simulink model "gm_sampleModel1666_2_sub"  (R2023a)
settings: Solver=VariableStepAuto  StartTime=0.0  StopTime=10.0  RelTol=1e-3
libraries: simulink x2
settings Model: Creator=user1  LastModifiedBy=user1
settings OptimizationCC: BlockReduction=off  ConditionallyExecuteInputs=off
settings DebuggingCC: InheritedTsInSrcMsg=none

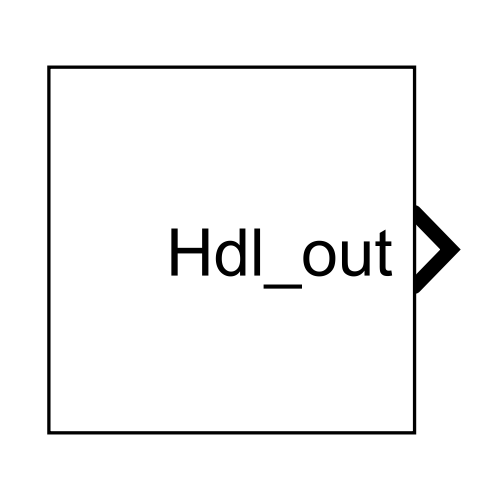
[thumbnail: Simulink's stored preview of the top-level diagram]
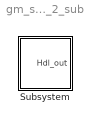
== system gm_sampleModel1666_2_sub ==
  Subsystem : Subsystem

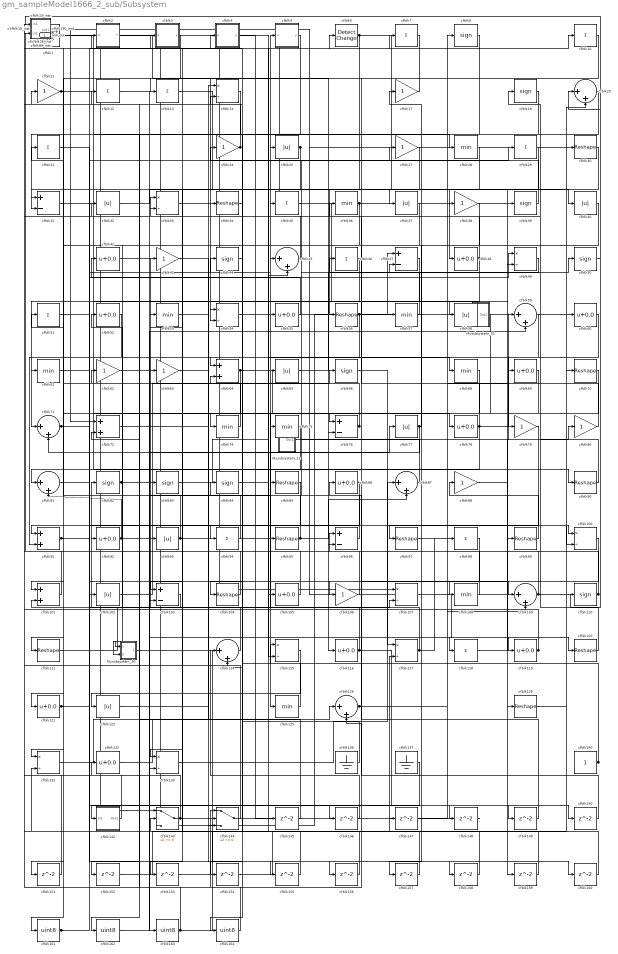
== system gm_sampleModel1666_2_sub/Subsystem ==
  Mysubsystem_12 : Subsystem
  Mysubsystem_30 : Subsystem
  Mysubsystem_31 : Subsystem
  cfblk1 : simulink/Logic and Bit Operations/Extract Bits  bitsToExtract=Upper half  numBits=8  bitIdxRange=[0 7]  outScalingMode=Preserve fixed-point scaling
      settings: LibrarySourceBlock=|
      | hdlsllib/Logic and Bit
      | Operations/Extract Bits
  cfblk{7,10,12..13,21,29,35,46,51,94,98,118} (12 alike) : Sum  Inputs=+  OutDataTypeStr=uint8
  cfblk{14,33,49,54,100,107,115,117,131,133} (10 alike) : Product  Inputs=*/  OutDataTypeStr=uint8  RndMeth=Zero  SaturateOnIntegerOverflow=on
  cfblk{64,72,91,101} (4 alike) : Sum  OutDataTypeStr=uint8
  cfblk{25,32,37,40,58,65,77,93,102,122} (10 alike) : Abs  OutDataTypeStr=uint8  SaturateOnIntegerOverflow=off
  cfblk{31,47,76,96,103} (5 alike) : Sum  Inputs=+-  OutDataTypeStr=uint8
  cfblk{30,34,56,70,85,90,95,97,99,104,111,120,129} (13 alike) : Reshape
  cfblk{42,48,52,55,60,69,78,86,92,105,116,119,121,132} (14 alike) : Bias  Bias=0.0  SaturateOnIntegerOverflow=off
  cfblk{11,17,24,27,38,43,62..63,79..80,88,106} (12 alike) : Gain  OutDataTypeStr=uint8
  cfblk{28,36,53,57,61,68,74..75,108,125} (10 alike) : MinMax  OutDataTypeStr=uint8
  cfblk{20,45,59,71,81,87,109,114,126} (9 alike) : Sum  Inputs=|++  OutDataTypeStr=uint8
  cfblk{8,19,39,44,50,66,82..84,110} (10 alike) : Signum
  cfblk112_inst : Subsystem
  cfblk113_inst : Subsystem
  cfblk124_inst : Subsystem
  cfblk128_inst : Subsystem
  cfblk130_inst : Subsystem
  cfblk136 : Ground
  cfblk137 : Ground
  cfblk140 : Constant  OutDataTypeStr=uint8  SampleTime=-1
  cfblk142 : Subsystem
  cfblk143 : Switch  OutDataTypeStr=uint8  SaturateOnIntegerOverflow=off  InputSameDT=off
  cfblk144 : Switch  OutDataTypeStr=uint8  SaturateOnIntegerOverflow=off  InputSameDT=off
  cfblk{145..160} (16 alike) : Delay  SampleTime=1
  cfblk15_inst : Subsystem
  cfblk{161..164} (4 alike) : DataTypeConversion  OutDataTypeStr=uint8  SaturateOnIntegerOverflow=off  RndMeth=Floor
  cfblk16_inst : Subsystem
  cfblk2 : Subsystem  mask(Detect Rise Positive){vinit=double(0), InputProcessing=Elements as channels (sample based), OutDataTypeStr=uint8}
      mask prompts: vinit "Simulink:masks:InitialCondition_MP"; InputProcessing "Simulink:masks:InputProcessing_MP"; OutDataTypeStr "Simulink:masks:OutputDataType_MP"
      mask help: Simulink:masks:DetectRisePositive_MD
      mask init:
      | InputProcessing = 'Elements as channels (sample based)';
      | OutDataTypeStr = 'uint8';
      | vinit = double(0);
      mask TypeOptions InputProcessing: Simulink:masks:ColumnsAsChannelsFrameBased | Simulink:masks:ElementsAsChannelsSampleBased
      mask TypeOptions OutDataTypeStr: Simulink:masks:uint8 | Simulink:masks:boolean
      mask Display: fprintf('U > 0\n&  NOT\nU/z > 0')
  cfblk26_inst : Subsystem
  cfblk3 : Subsystem  mask(Compare To Zero){relop=<=, OutDataTypeStr=uint8, ZeroCross=on}
      mask prompts: relop "Simulink:masks:Operator_MP"; OutDataTypeStr "Simulink:masks:OutputDataType_MP"; ZeroCross "Simulink:masks:EnableZerocrossingDetection_MP"
      mask help: Simulink:masks:CompareToZero_MD
      mask init:
      | OutDataTypeStr = 'uint8';
      | ZeroCross = 'on';
      | blkName = 'sampleModel1666_2_sub/Subsystem/cfblk3';
      | relop = '<=';
      | setValue = 'fixdt(0, 8)';
      mask TypeOptions relop: == | ~= | < | <= | >= | >
      mask TypeOptions OutDataTypeStr: Simulink:masks:uint8 | Simulink:masks:boolean
      mask Callback ZeroCross: sl('zeroCrossEnable', gcbh);
      mask Display: disp([relop,' 0'])
  cfblk4 : Subsystem  mask(Compare To Constant){relop=<=, const=double(3), OutDataTypeStr=uint8, ZeroCross=on}
      mask prompts: relop "Simulink:masks:Operator_MP"; const "Simulink:masks:ConstantValue_MP"; OutDataTypeStr "Simulink:masks:OutputDataType_MP"; ZeroCross "Simulink:masks:EnableZerocrossingDetection_MP"
      mask help: Simulink:masks:CompareToConstant_MD
      mask init:
      | OutDataTypeStr = 'uint8';
      | ZeroCross = 'on';
      | blkName = 'sampleModel1666_2_sub/Subsystem/cfblk4';
      | const = double(3);
      | const_str = '3.0';
      | const_val = double(3);
      | relop = '<=';
      | setValue = 'fixdt(0, 8)';
      | str = '<= 3';
      mask TypeOptions relop: == | ~= | < | <= | >= | >
      mask TypeOptions OutDataTypeStr: Simulink:masks:uint8 | Simulink:masks:boolean
      mask Callback ZeroCross: sl('zeroCrossEnable', gcbh);
      mask Display: disp(str)
  cfblk5 : Subsystem  mask(Compare To Constant){relop=<=, const=double(3), OutDataTypeStr=uint8, ZeroCross=on}
      mask prompts: relop "Simulink:masks:Operator_MP"; const "Simulink:masks:ConstantValue_MP"; OutDataTypeStr "Simulink:masks:OutputDataType_MP"; ZeroCross "Simulink:masks:EnableZerocrossingDetection_MP"
      mask help: Simulink:masks:CompareToConstant_MD
      mask init:
      | OutDataTypeStr = 'uint8';
      | ZeroCross = 'on';
      | blkName = 'sampleModel1666_2_sub/Subsystem/cfblk5';
      | const = double(3);
      | const_str = '3.0';
      | const_val = double(3);
      | relop = '<=';
      | setValue = 'fixdt(0, 8)';
      | str = '<= 3';
      mask TypeOptions relop: == | ~= | < | <= | >= | >
      mask TypeOptions OutDataTypeStr: Simulink:masks:uint8 | Simulink:masks:boolean
      mask Callback ZeroCross: sl('zeroCrossEnable', gcbh);
      mask Display: disp(str)
  cfblk6 : simulink/Logic and Bit Operations/Detect Change  vinit=0  OutDataTypeStr=uint8
      settings: LibrarySourceBlock=|
      | hdlsllib/Logic and Bit
      | Operations/Detect
      | Change
  cfblk89_inst : Subsystem
  Hdl_out : Outport  OutDataTypeStr=uint8  SampleTime=1
  wires:
  Mysubsystem_12/1(Out1) -> cfblk59/1
  Mysubsystem_30/1(Out1) -> cfblk156/1
  Mysubsystem_31/1(Out1) -> cfblk125/1
  cfblk1/1 -> cfblk58/1, cfblk28/1
  cfblk10/1 -> cfblk54/2
  cfblk100/1 -> cfblk144/1
  cfblk101/1 -> cfblk130_inst/2(in2)
  cfblk102/1 -> cfblk66/1
  cfblk103/1 -> cfblk82/1
  cfblk104/1 -> cfblk43/1
  cfblk105/1 -> cfblk4/1(u)
  cfblk106/1 -> cfblk33/1
  cfblk107/1 -> cfblk119/1
  cfblk108/1 -> cfblk96/1
  cfblk109/1 -> cfblk128_inst/1(in1), cfblk5/1(u)
  cfblk11/1 -> cfblk90/1, cfblk76/1
  cfblk110/1 -> cfblk112_inst/2(in2), cfblk62/1
  cfblk111/1 -> cfblk93/1
  cfblk112_inst/1(out1) -> cfblk145/1
  cfblk113_inst/1(out1) -> cfblk30/1
  cfblk114/1 -> cfblk53/1
  cfblk115/1 -> cfblk122/1
  cfblk116/1 -> cfblk55/1, cfblk150/1
  cfblk117/1 -> cfblk52/1, cfblk98/1
  cfblk118/1 -> cfblk80/1
  cfblk119/1 -> cfblk124_inst/1(in1), cfblk63/1
  cfblk12/1 -> cfblk163/1
  cfblk120/1 -> cfblk33/2
  cfblk121/1 -> cfblk149/1, cfblk148/1, cfblk107/2
  cfblk122/1 -> cfblk34/1
  cfblk124_inst/1(out1) -> cfblk57/1
  cfblk125/1 -> cfblk115/1
  cfblk126/1 -> cfblk86/1, cfblk8/1
  cfblk128_inst/1(out1) -> cfblk110/1, Hdl_out/1
  cfblk129/1 -> cfblk70/1
  cfblk13/1 -> cfblk56/1
  cfblk130_inst/1(out1) -> cfblk143/1
  cfblk131/1 -> cfblk14/1
  cfblk132/1 -> cfblk126/1
  cfblk133/1 -> cfblk87/1
  cfblk136/1 -> cfblk14/2
  cfblk137/1 -> cfblk142/1(In1)
  cfblk14/1 -> cfblk162/1
  cfblk140/1 -> cfblk92/1, cfblk128_inst/2(in2), cfblk2/1(U)
  cfblk142/1(Out1) -> cfblk15_inst/1(in1)
  cfblk143/1 -> cfblk83/1, cfblk132/1
  cfblk144/1 -> cfblk89_inst/1(in1)
  cfblk145/1 -> cfblk72/2
  cfblk146/1 -> cfblk114/1
  cfblk147/1 -> cfblk109/2
  cfblk148/1 -> cfblk1/1
  cfblk149/1 -> cfblk101/2
  cfblk15_inst/1(out1) -> cfblk72/1
  cfblk150/1 -> cfblk126/2
  cfblk151/1 -> cfblk130_inst/1(in1)
  cfblk152/1 -> cfblk45/2
  cfblk153/1 -> cfblk117/2
  cfblk154/1 -> cfblk20/2
  cfblk155/1 -> cfblk64/2
  cfblk156/1 -> cfblk113_inst/1(in1)
  cfblk157/1 -> cfblk103/2
  cfblk158/1 -> cfblk26_inst/2(in2)
  cfblk159/1 -> cfblk143/2
  cfblk16_inst/1(out1) -> cfblk107/1
  cfblk160/1 -> cfblk131/2
  cfblk161/1 -> cfblk44/1, cfblk49/1
  cfblk162/1 -> cfblk85/1
  cfblk163/1 -> cfblk113_inst/2(in2), cfblk147/1
  cfblk164/1 -> cfblk12/1
  cfblk17/1 -> cfblk13/1
  cfblk19/1 -> cfblk31/2
  cfblk2/1(Y) -> cfblk76/2
  cfblk20/1 -> cfblk121/1
  cfblk21/1 -> cfblk102/1
  cfblk24/1 -> cfblk15_inst/2(in2), cfblk124_inst/2(in2)
  cfblk25/1 -> cfblk153/1, cfblk152/1
  cfblk26_inst/1(out1) -> cfblk95/1, cfblk39/1, cfblk16_inst/1(in1)
  cfblk27/1 -> cfblk37/1
  cfblk28/1 -> cfblk115/2
  cfblk29/1 -> cfblk48/1
  cfblk3/1(y) -> cfblk101/1
  cfblk30/1 -> cfblk91/1
  cfblk31/1 -> cfblk116/1
  cfblk32/1 -> cfblk38/1
  cfblk33/1 -> cfblk40/1
  cfblk34/1 -> cfblk74/1
  cfblk35/1 -> cfblk129/1
  cfblk36/1 -> cfblk111/1, Mysubsystem_30/1(In1)
  cfblk37/1 -> cfblk114/2
  cfblk38/1 -> cfblk54/1
  cfblk39/1 -> cfblk24/1
  cfblk4/1(y) -> cfblk106/1
  cfblk40/1 -> cfblk97/1
  cfblk42/1 -> cfblk75/1
  cfblk43/1 -> cfblk144/2
  cfblk44/1 -> cfblk164/1
  cfblk45/1 -> cfblk21/1
  cfblk46/1 -> cfblk71/1
  cfblk47/1 -> cfblk133/1
  cfblk48/1 -> cfblk89_inst/2(in2), cfblk154/1
  cfblk49/1 -> cfblk47/2
  cfblk5/1(y) -> cfblk104/1
  cfblk50/1 -> cfblk20/1
  cfblk51/1 -> cfblk29/1
  cfblk52/1 -> cfblk61/1
  cfblk53/1 -> cfblk120/1
  cfblk54/1 -> cfblk68/1
  cfblk55/1 -> cfblk42/1
  cfblk56/1 -> cfblk47/1, Mysubsystem_30/2(In2)
  cfblk57/1 -> cfblk32/1
  cfblk58/1 -> cfblk60/1, cfblk143/3
  cfblk59/1 -> cfblk79/1
  cfblk6/1 -> cfblk99/1, cfblk64/1, cfblk49/2
  cfblk60/1 -> cfblk91/2
  cfblk61/1 -> cfblk109/1
  cfblk62/1 -> cfblk78/1
  cfblk63/1 -> cfblk158/1
  cfblk64/1 -> cfblk96/2, cfblk144/3
  cfblk65/1 -> cfblk50/1
  cfblk66/1 -> cfblk117/1
  cfblk68/1 -> cfblk103/1
  cfblk69/1 -> cfblk81/1
  cfblk7/1 -> cfblk146/1
  cfblk70/1 -> cfblk151/1
  cfblk71/1 -> cfblk100/1, cfblk7/1
  cfblk72/1 -> cfblk27/1
  cfblk74/1 -> cfblk3/1(u)
  cfblk75/1 -> cfblk133/2
  cfblk76/1 -> cfblk25/1, cfblk51/1
  cfblk77/1 -> cfblk71/2, cfblk17/1
  cfblk78/1 -> cfblk131/1, cfblk100/2, cfblk46/1
  cfblk79/1 -> cfblk157/1
  cfblk8/1 -> cfblk31/1
  cfblk80/1 -> cfblk36/1
  cfblk81/1 -> cfblk45/1
  cfblk82/1 -> cfblk59/2, cfblk118/1
  cfblk83/1 -> cfblk10/1
  cfblk84/1 -> cfblk105/1
  cfblk85/1 -> cfblk161/1
  cfblk86/1 -> cfblk94/1
  cfblk87/1 -> cfblk35/1
  cfblk88/1 -> cfblk159/1
  cfblk89_inst/1(out1) -> cfblk112_inst/1(in1)
  cfblk90/1 -> cfblk19/1
  cfblk91/1 -> cfblk160/1, cfblk6/1
  cfblk92/1 -> cfblk84/1, cfblk81/2, cfblk77/1
  cfblk93/1 -> cfblk155/1, cfblk11/1
  cfblk94/1 -> cfblk26_inst/1(in1)
  cfblk95/1 -> cfblk87/2, cfblk16_inst/2(in2)
  cfblk96/1 -> cfblk65/1
  cfblk97/1 -> cfblk69/1
  cfblk98/1 -> cfblk108/1
  cfblk99/1 -> cfblk88/1

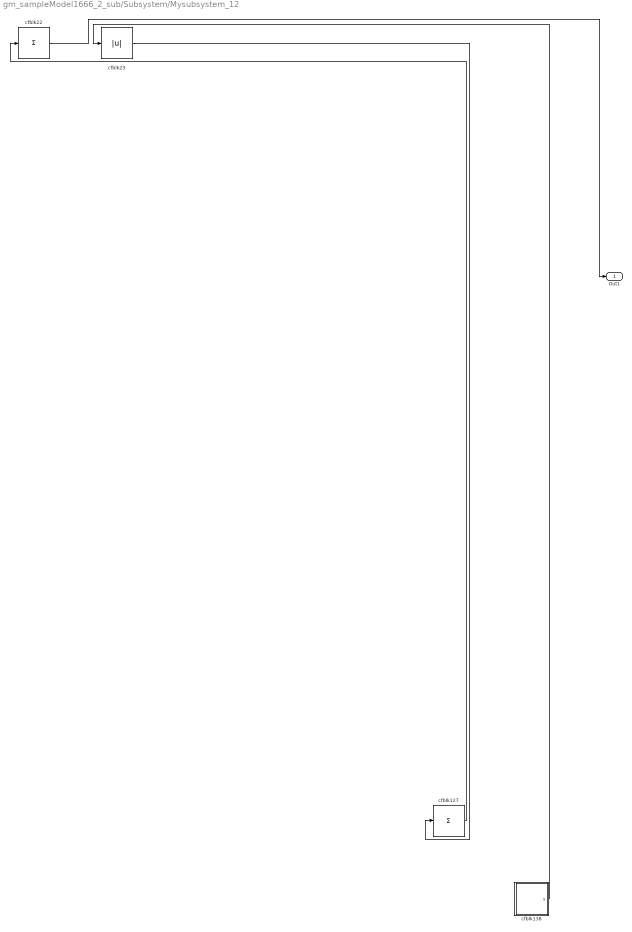
== system gm_sampleModel1666_2_sub/Subsystem/Mysubsystem_12 ==
  cfblk127 : Sum  Inputs=+
  cfblk138 : Subsystem  mask(Counter Free-Running){NumBits=double(16), tsamp=double(-1)}
      mask prompts: NumBits "Simulink:masks:NumberOfBits_MP"; tsamp "Simulink:masks:SampleTime_MP"
      mask help: Simulink:masks:CounterFreeRunning_MD
  cfblk22 : Sum  Inputs=+
  cfblk23 : Abs  SaturateOnIntegerOverflow=off
  Out1 : Outport  SampleTime=1
  wires:
  cfblk127/1 -> cfblk22/1
  cfblk138/1(y) -> cfblk23/1
  cfblk22/1 -> Out1/1
  cfblk23/1 -> cfblk127/1

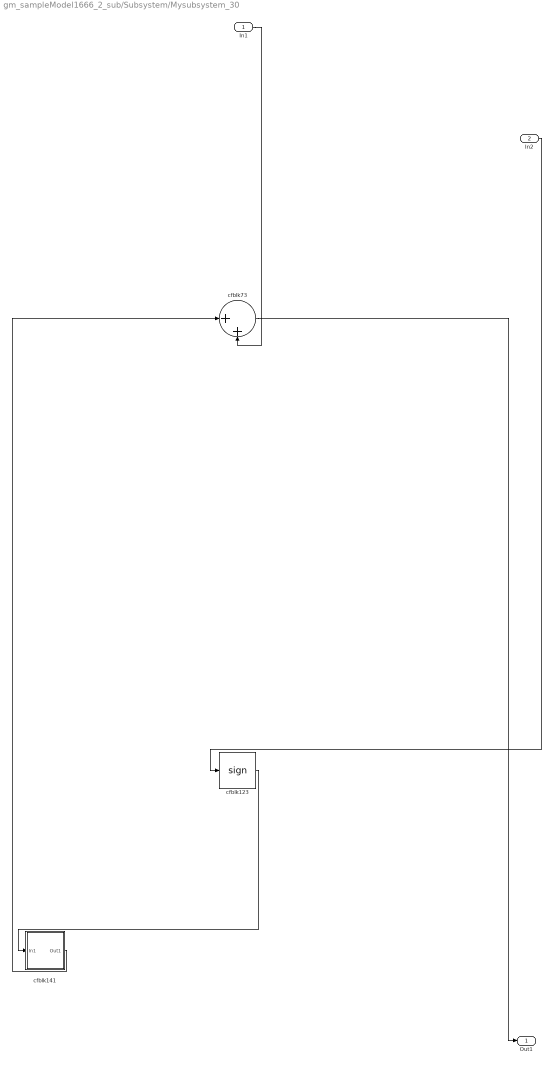
== system gm_sampleModel1666_2_sub/Subsystem/Mysubsystem_30 ==
  In1 : Inport  OutDataTypeStr=uint8  PortDimensions=1  SampleTime=1
  In2 : Inport  Port=2  OutDataTypeStr=uint8  PortDimensions=1  SampleTime=1
  cfblk123 : Signum
  cfblk141 : Subsystem
  cfblk73 : Sum  Inputs=|++
  Out1 : Outport  SampleTime=1
  wires:
  In1/1 -> cfblk73/2
  In2/1 -> cfblk123/1
  cfblk123/1 -> cfblk141/1(In1)
  cfblk141/1(Out1) -> cfblk73/1
  cfblk73/1 -> Out1/1

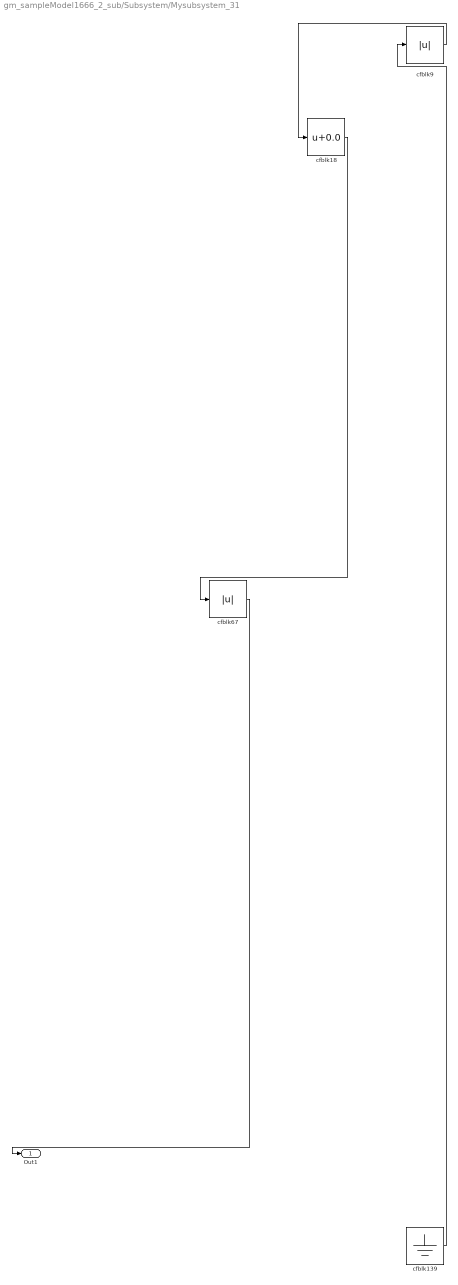
== system gm_sampleModel1666_2_sub/Subsystem/Mysubsystem_31 ==
  cfblk139 : Ground
  cfblk18 : Bias  Bias=0.0  SaturateOnIntegerOverflow=off
  cfblk67 : Abs  SaturateOnIntegerOverflow=off
  cfblk9 : Abs  SaturateOnIntegerOverflow=off
  Out1 : Outport  SampleTime=1
  wires:
  cfblk139/1 -> cfblk9/1
  cfblk18/1 -> cfblk67/1
  cfblk67/1 -> Out1/1
  cfblk9/1 -> cfblk18/1

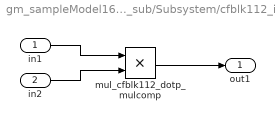
== system gm_sampleModel1666_2_sub/Subsystem/cfblk112_inst ==
  in1 : Inport  OutDataTypeStr=uint8  SampleTime=1
  in2 : Inport  Port=2  OutDataTypeStr=uint8  SampleTime=1
  mul_cfblk112_dotp_mulcomp : Product  Inputs=**  OutDataTypeStr=uint8  SampleTime=1
  out1 : Outport  OutDataTypeStr=uint8  SampleTime=1
  wires:
  in1/1 -> mul_cfblk112_dotp_mulcomp/1
  in2/1 -> mul_cfblk112_dotp_mulcomp/2
  mul_cfblk112_dotp_mulcomp/1 -> out1/1

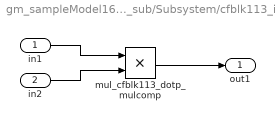
== system gm_sampleModel1666_2_sub/Subsystem/cfblk113_inst ==
  in1 : Inport  OutDataTypeStr=uint8  SampleTime=1
  in2 : Inport  Port=2  OutDataTypeStr=uint8  SampleTime=1
  mul_cfblk113_dotp_mulcomp : Product  Inputs=**  OutDataTypeStr=uint8  SampleTime=1
  out1 : Outport  OutDataTypeStr=uint8  SampleTime=1
  wires:
  in1/1 -> mul_cfblk113_dotp_mulcomp/1
  in2/1 -> mul_cfblk113_dotp_mulcomp/2
  mul_cfblk113_dotp_mulcomp/1 -> out1/1

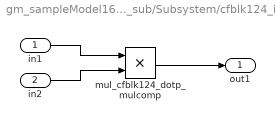
== system gm_sampleModel1666_2_sub/Subsystem/cfblk124_inst ==
  in1 : Inport  OutDataTypeStr=uint8  SampleTime=1
  in2 : Inport  Port=2  OutDataTypeStr=uint8  SampleTime=1
  mul_cfblk124_dotp_mulcomp : Product  Inputs=**  OutDataTypeStr=uint8  SampleTime=1
  out1 : Outport  OutDataTypeStr=uint8  SampleTime=1
  wires:
  in1/1 -> mul_cfblk124_dotp_mulcomp/1
  in2/1 -> mul_cfblk124_dotp_mulcomp/2
  mul_cfblk124_dotp_mulcomp/1 -> out1/1

== system gm_sampleModel1666_2_sub/Subsystem/cfblk128_inst ==
  in1 : Inport  OutDataTypeStr=uint8  SampleTime=1
  in2 : Inport  Port=2  OutDataTypeStr=uint8  SampleTime=1
  mul_cfblk128_dotp_mulcomp : Product  Inputs=**  OutDataTypeStr=uint8  SampleTime=1
  out1 : Outport  OutDataTypeStr=uint8  SampleTime=1
  wires:
  in1/1 -> mul_cfblk128_dotp_mulcomp/1
  in2/1 -> mul_cfblk128_dotp_mulcomp/2
  mul_cfblk128_dotp_mulcomp/1 -> out1/1

== system gm_sampleModel1666_2_sub/Subsystem/cfblk130_inst ==
  in1 : Inport  OutDataTypeStr=uint8  SampleTime=1
  in2 : Inport  Port=2  OutDataTypeStr=uint8  SampleTime=1
  mul_cfblk130_dotp_mulcomp : Product  Inputs=**  OutDataTypeStr=uint8  SampleTime=1
  out1 : Outport  OutDataTypeStr=uint8  SampleTime=1
  wires:
  in1/1 -> mul_cfblk130_dotp_mulcomp/1
  in2/1 -> mul_cfblk130_dotp_mulcomp/2
  mul_cfblk130_dotp_mulcomp/1 -> out1/1

== system gm_sampleModel1666_2_sub/Subsystem/cfblk142 ==
  In1 : Inport  OutDataTypeStr=uint8  PortDimensions=1  SampleTime=1
  Out1 : Outport  SampleTime=1
  wires:
  In1/1 -> Out1/1

== system gm_sampleModel1666_2_sub/Subsystem/cfblk15_inst ==
  in1 : Inport  OutDataTypeStr=uint8  SampleTime=1
  in2 : Inport  Port=2  OutDataTypeStr=uint8  SampleTime=1
  mul_cfblk15_dotp_mulcomp : Product  Inputs=**  OutDataTypeStr=uint8  SampleTime=1
  out1 : Outport  OutDataTypeStr=uint8  SampleTime=1
  wires:
  in1/1 -> mul_cfblk15_dotp_mulcomp/1
  in2/1 -> mul_cfblk15_dotp_mulcomp/2
  mul_cfblk15_dotp_mulcomp/1 -> out1/1

== system gm_sampleModel1666_2_sub/Subsystem/cfblk16_inst ==
  in1 : Inport  OutDataTypeStr=uint8  SampleTime=1
  in2 : Inport  Port=2  OutDataTypeStr=uint8  SampleTime=1
  mul_cfblk16_dotp_mulcomp : Product  Inputs=**  OutDataTypeStr=uint8  SampleTime=1
  out1 : Outport  OutDataTypeStr=uint8  SampleTime=1
  wires:
  in1/1 -> mul_cfblk16_dotp_mulcomp/1
  in2/1 -> mul_cfblk16_dotp_mulcomp/2
  mul_cfblk16_dotp_mulcomp/1 -> out1/1

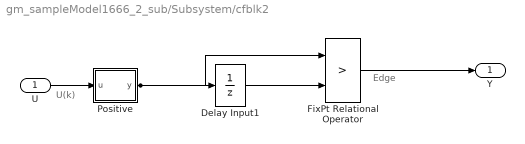
== system gm_sampleModel1666_2_sub/Subsystem/cfblk2 ==
  note: U(k)
  note: Edge
  U : Inport  OutDataTypeStr=uint8  SampleTime=1
  Delay Input1 : UnitDelay  Description=Store in Global RAM  DisableCoverage=on  InitialCondition=vinit  SampleTime=-1  HasFrameUpgradeWarning=on
  FixPt Relational Operator : RelationalOperator  Operator=>  OutDataTypeStr=fixdt(0, 8)  ZeroCross=off  InputSameDT=off
  Positive : Subsystem  mask(Compare To Zero){relop=>, OutDataTypeStr=boolean, ZeroCross=off}
      mask prompts: relop "Simulink:masks:Operator_MP"; OutDataTypeStr "Simulink:masks:OutputDataType_MP"; ZeroCross "Simulink:masks:EnableZerocrossingDetection_MP"
      mask help: Simulink:masks:CompareToZero_MD
      mask init:
      | OutDataTypeStr = 'boolean';
      | ZeroCross = 'off';
      | blkName = 'sampleModel1666_2_sub/Subsystem/cfblk2/Positive';
      | relop = '>';
      | setValue = 'boolean';
      mask TypeOptions relop: == | ~= | < | <= | >= | >
      mask TypeOptions OutDataTypeStr: Simulink:masks:uint8 | Simulink:masks:boolean
      mask Callback ZeroCross: sl('zeroCrossEnable', gcbh);
      mask Display: disp([relop,' 0'])
  Y : Outport  SampleTime=1
  wires:
  U/1 -> Positive/1(u)
  Delay Input1/1 -> FixPt Relational Operator/2
  FixPt Relational Operator/1 -> Y/1
  Positive/1(y) -> FixPt Relational Operator/1, Delay Input1/1

== system gm_sampleModel1666_2_sub/Subsystem/cfblk26_inst ==
  in1 : Inport  OutDataTypeStr=uint8  SampleTime=1
  in2 : Inport  Port=2  OutDataTypeStr=uint8  SampleTime=1
  mul_cfblk26_dotp_mulcomp : Product  Inputs=**  OutDataTypeStr=uint8  SampleTime=1
  out1 : Outport  OutDataTypeStr=uint8  SampleTime=1
  wires:
  in1/1 -> mul_cfblk26_dotp_mulcomp/1
  in2/1 -> mul_cfblk26_dotp_mulcomp/2
  mul_cfblk26_dotp_mulcomp/1 -> out1/1

== system gm_sampleModel1666_2_sub/Subsystem/cfblk3 ==
  u : Inport  OutDataTypeStr=uint8  SampleTime=1
  Compare : RelationalOperator  Operator=<=  OutDataTypeStr=fixdt(0, 8)
  Constant : Constant  DisableCoverage=on  Value=0  OutDataTypeStr=Inherit: Inherit via back propagation  SampleTime=-1  PreserveConstantTs=on
  y : Outport  SampleTime=1
  wires:
  u/1 -> Compare/1
  Compare/1 -> y/1
  Constant/1 -> Compare/2

== system gm_sampleModel1666_2_sub/Subsystem/cfblk4 ==
  u : Inport  OutDataTypeStr=uint8  SampleTime=1
  Compare : RelationalOperator  Operator=<=  OutDataTypeStr=fixdt(0, 8)
  Constant : Constant  DisableCoverage=on  Value=const  OutDataTypeStr=Inherit: Inherit via back propagation  SampleTime=-1
  y : Outport  SampleTime=1
  wires:
  u/1 -> Compare/1
  Compare/1 -> y/1
  Constant/1 -> Compare/2

== system gm_sampleModel1666_2_sub/Subsystem/cfblk5 ==
  u : Inport  OutDataTypeStr=uint8  SampleTime=1
  Compare : RelationalOperator  Operator=<=  OutDataTypeStr=fixdt(0, 8)
  Constant : Constant  DisableCoverage=on  Value=const  OutDataTypeStr=Inherit: Inherit via back propagation  SampleTime=-1
  y : Outport  SampleTime=1
  wires:
  u/1 -> Compare/1
  Compare/1 -> y/1
  Constant/1 -> Compare/2

== system gm_sampleModel1666_2_sub/Subsystem/cfblk89_inst ==
  in1 : Inport  OutDataTypeStr=uint8  SampleTime=1
  in2 : Inport  Port=2  OutDataTypeStr=uint8  SampleTime=1
  mul_cfblk89_dotp_mulcomp : Product  Inputs=**  OutDataTypeStr=uint8  SampleTime=1
  out1 : Outport  OutDataTypeStr=uint8  SampleTime=1
  wires:
  in1/1 -> mul_cfblk89_dotp_mulcomp/1
  in2/1 -> mul_cfblk89_dotp_mulcomp/2
  mul_cfblk89_dotp_mulcomp/1 -> out1/1

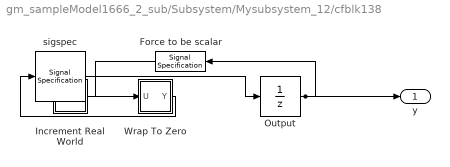
== system gm_sampleModel1666_2_sub/Subsystem/Mysubsystem_12/cfblk138 ==
  Force to be scalar : SignalSpecification  DisableCoverage=on  Dimensions=1
  Increment Real World : Subsystem  mask(Real World Value Increment){}
      mask help: Simulink:masks:RealWorldValueIncrement_MD
      mask Display: disp('V++')
  Output : UnitDelay  InitialCondition=0.0  SampleTime=tsamp  HasFrameUpgradeWarning=on
  Wrap To Zero : Subsystem  mask(Wrap To Zero){Threshold=double(65535)}
      mask prompts: Threshold "Simulink:masks:Threshold_MP"
      mask help: Simulink:masks:WrapToZero_MD
  sigspec : SignalSpecification  OutDataTypeStr=uint16  Dimensions=1
  y : Outport  SampleTime=1
  wires:
  Force to be scalar/1 -> Increment Real World/1(u)
  Increment Real World/1(y) -> Wrap To Zero/1(U)
  Output/1 -> Force to be scalar/1, y/1
  Wrap To Zero/1(Y) -> sigspec/1
  sigspec/1 -> Output/1

== system gm_sampleModel1666_2_sub/Subsystem/Mysubsystem_30/cfblk141 ==
  In1 : Inport  OutDataTypeStr=uint8  PortDimensions=1  SampleTime=1
  Out1 : Outport  SampleTime=1
  wires:
  In1/1 -> Out1/1

== system gm_sampleModel1666_2_sub/Subsystem/cfblk2/Positive ==
  u : Inport  OutDataTypeStr=uint8  SampleTime=1
  Compare : RelationalOperator  Operator=>  OutDataTypeStr=boolean  ZeroCross=off
  Constant : Constant  DisableCoverage=on  Value=0  OutDataTypeStr=Inherit: Inherit via back propagation  SampleTime=-1  PreserveConstantTs=on
  y : Outport  SampleTime=1
  wires:
  u/1 -> Compare/1
  Compare/1 -> y/1
  Constant/1 -> Compare/2

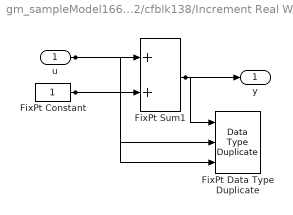
== system gm_sampleModel1666_2_sub/Subsystem/Mysubsystem_12/cfblk138/Increment Real World ==
  u : Inport  OutDataTypeStr=uint16  SampleTime=1
  FixPt Constant : Constant  DisableCoverage=on  OutDataTypeStr=Inherit: Inherit via back propagation  SampleTime=-1
  FixPt Data Type Duplicate : DataTypeDuplicate  DisableCoverage=on  NumInputPorts=3
  FixPt Sum1 : Sum  InputSameDT=on  OutDataTypeStr=Inherit: Inherit via back propagation  LockScale=on
  y : Outport  SampleTime=1
  wires:
  u/1 -> FixPt Sum1/1, FixPt Data Type Duplicate/2
  FixPt Constant/1 -> FixPt Sum1/2, FixPt Data Type Duplicate/3
  FixPt Sum1/1 -> FixPt Data Type Duplicate/1, y/1

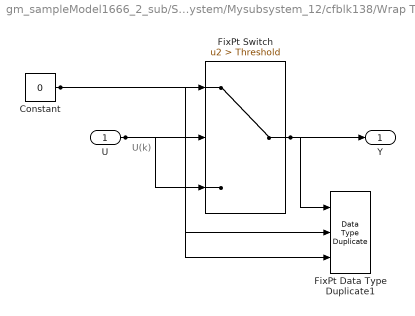
== system gm_sampleModel1666_2_sub/Subsystem/Mysubsystem_12/cfblk138/Wrap To Zero ==
  note: U(k)
  U : Inport  OutDataTypeStr=uint16  SampleTime=1
  Constant : Constant  DisableCoverage=on  Value=0  OutDataTypeStr=Inherit: Inherit via back propagation  SampleTime=-1
  FixPt Data Type Duplicate1 : DataTypeDuplicate  DisableCoverage=on  NumInputPorts=3
  FixPt Switch : Switch  Criteria=u2 > Threshold  Threshold=Threshold  OutDataTypeStr=Inherit: Inherit via back propagation  ZeroCross=off  SaturateOnIntegerOverflow=off  InputSameDT=off
  Y : Outport  SampleTime=1
  wires:
  U/1 -> FixPt Switch/3, FixPt Switch/2, FixPt Data Type Duplicate1/2
  Constant/1 -> FixPt Switch/1, FixPt Data Type Duplicate1/3
  FixPt Switch/1 -> FixPt Data Type Duplicate1/1, Y/1
